simulink model "test_state"  (R2022b)
settings: Solver=VariableStepAuto  StartTime=0.0  StopTime=10.0  RelTol=1e-3
settings Model: Creator=KenYoshioka  LastModifiedBy=KenYoshioka

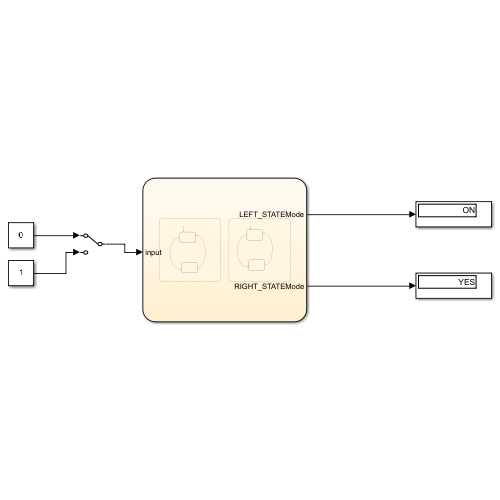
[thumbnail: Simulink's stored preview of the top-level diagram]
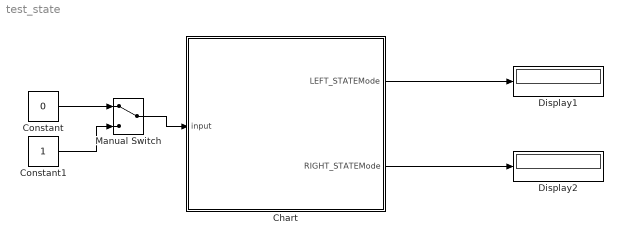
== system test_state ==
  Chart : Stateflow chart  TreatAsAtomicUnit=on
  Constant : Constant  Value=0
  Constant1 : Constant
  Display1 : Display
  Display2 : Display
  Manual Switch : ManualSwitch
  wires:
  Manual Switch/1 -> Chart/1(input)
  Constant/1 -> Manual Switch/1
  Constant1/1 -> Manual Switch/2
  Chart/1(" LEFT_STATEMode") -> Display1/1
  Chart/2(" RIGHT_STATEMode") -> Display2/1

== stateflow chart test_state/Chart ==
  state LEFT_STATE [parallel]
    settings: executionOrder=1
    state ON
    state OFF
    (default) -> ON
    OFF -> ON : [~input]
    ON -> OFF : [input]
  state RIGHT_STATE [parallel]
    settings: executionOrder=2
    state YES
    state NO
    (default) -> YES
    NO -> YES : [~input]
    YES -> NO : [input]
  data: input input; LEFT_STATEMode output Enum: LEFT_STATEModeType; RIGHT_STATEMode output Enum: RIGHT_STATEModeType
